simulink model "Lab3minge"  (R2013b)
settings: Solver=ode45  StartTime=0.0  StopTime=10.0  RelTol=1e-3
settings Model: Creator=User  LastModifiedBy=User
settings ConfigurationSet: Description=SimMechanics 2G

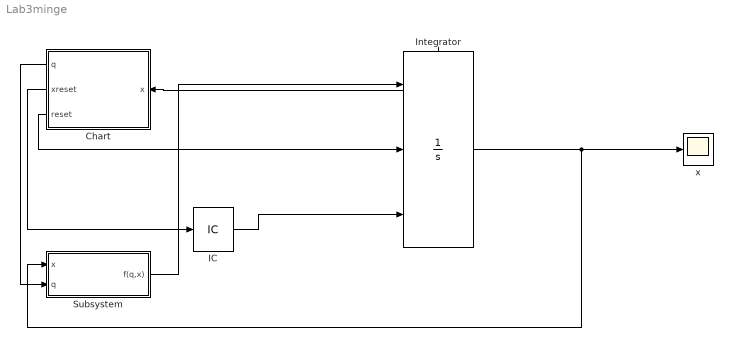
== system Lab3minge ==
  Chart : Stateflow chart  TreatAsAtomicUnit=on
  IC : InitialCondition  Value=[10;5]
  Integrator : Integrator  ExternalReset=rising  InitialConditionSource=external  LimitOutput=on  LowerSaturationLimit=[0;-inf]  ShowStatePort=on
  Subsystem : Subsystem
  x : Scope
  wires:
  Integrator/1 -> Subsystem/1(x), x/1
  Integrator/State -> Chart/1(x)
  Chart/1(q) -> Subsystem/2(q)
  Subsystem/1(f(q,x)) -> Integrator/1
  Chart/2(xreset) -> IC/1
  IC/1 -> Integrator/3
  Chart/3(reset) -> Integrator/2

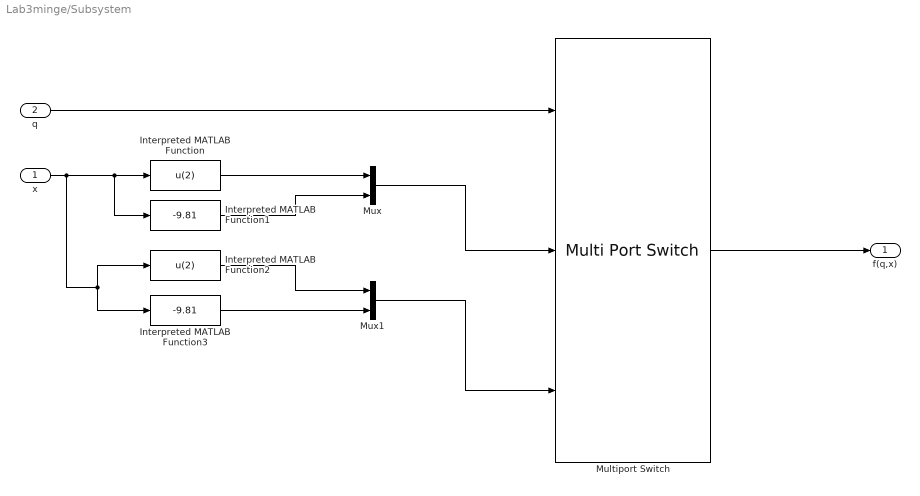
== system Lab3minge/Subsystem ==
  x : Inport
  q : Inport  Port=2
  Interpreted MATLAB Function : MATLABFcn  MATLABFcn=u(2)
  Interpreted MATLAB Function1 : MATLABFcn  MATLABFcn=-9.81
  Interpreted MATLAB Function2 : MATLABFcn  MATLABFcn=u(2)
  Interpreted MATLAB Function3 : MATLABFcn  MATLABFcn=-9.81
  Multiport Switch : MultiPortSwitch  Inputs=2
  Mux : Mux  Inputs=2
  Mux1 : Mux  Inputs=2
  f(q,x) : Outport
  wires:
  q/1 -> Multiport Switch/1
  Multiport Switch/1 -> f(q,x)/1
  Mux/1 -> Multiport Switch/2
  Mux1/1 -> Multiport Switch/3
  Interpreted MATLAB Function/1 -> Mux/1
  Interpreted MATLAB Function1/1 -> Mux/2
  Interpreted MATLAB Function2/1 -> Mux1/1
  Interpreted MATLAB Function3/1 -> Mux1/2
  x/1 -> Interpreted MATLAB Function3/1, Interpreted MATLAB Function2/1, Interpreted MATLAB Function1/1, Interpreted MATLAB Function/1

== stateflow chart Lab3minge/Chart ==
  state fall
    entry:q=1;
  fall -> fall : [x[1]<=0&&x[2]<0]/xreset[1]=x[1];xreset[2]=-0.4*x[2];reset
  (default) -> fall
  data: x input size=2; q output double; xreset output double size=2
  events: reset output EITHER_EDGE_EVENT
